simulink library "mfeval_STI_LIB"  (R2026a)
settings: Solver=ode45
undefined symbols (not defined in the file or in its folder): parameterStruct, userDynamics
libraries: sharedtransform x4, sharedutil x2, mfeval_CPI_LIB x1
Description:
  | Copyright 2020-2026 The MathWorks, Inc.
settings Model: Creator=MFURLANT  LastModifiedBy=smiller
settings DataIOCC: SaveFormat=StructureWithTime
settings HardwareCC: ProdHWDeviceType=Specified

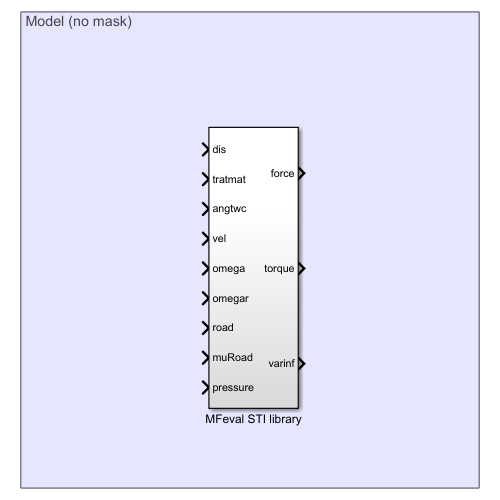
[thumbnail: Simulink's stored preview of the top-level diagram]
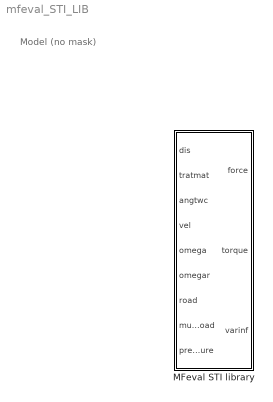
== system mfeval_STI_LIB ==
  note: Model (no mask)
  MFeval STI library : Subsystem

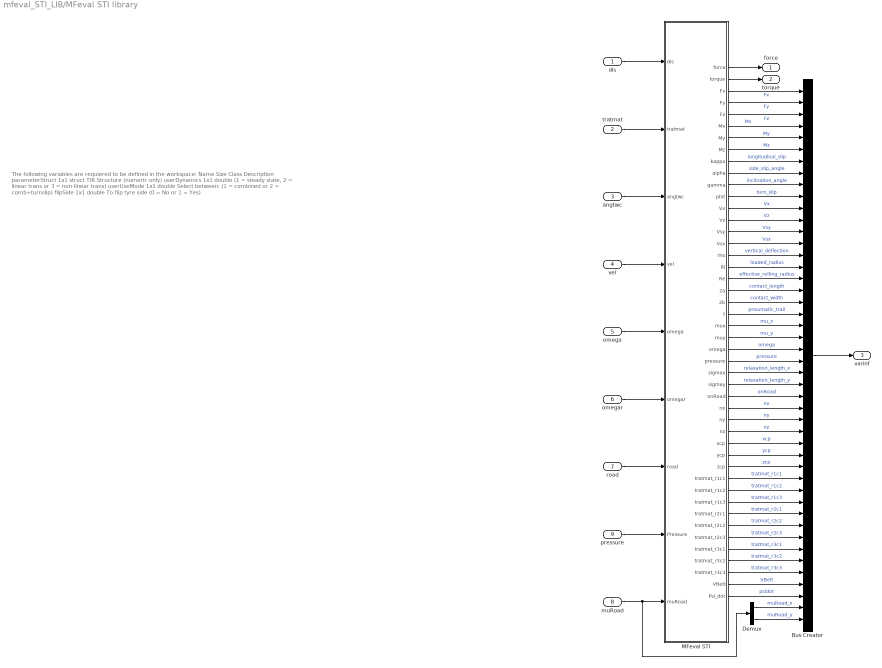
== system mfeval_STI_LIB/MFeval STI library ==
  note: The following variables are requiered to be defined in the workspace:
      |
      | Name
      | Size
      | Class
      | Description
      |
      | parameterStruct
      | 1x1
      | struct
      | TIR Structure (numeric only)
      |
      | userDynamics
      | 1x1
      | double
      | (1 = steady state, 2 = linear trans or 3 = non-linear trans)
      |
      | userUseMode
      | 1x1
      | double
      | Select between: (1 = combined or 2 = comb+turnslip)
      |
      | flipSide
      | 1x1
      | double
      | To flip tyre side (0 = No or 1 = Yes)
  dis : Inport
  tratmat : Inport  Port=2
  angtwc : Inport  Port=3
  vel : Inport  Port=4
  omega : Inport  Port=5
  omegar : Inport  Port=6
  road : Inport  Port=7
  muRoad : Inport  Port=8
  pressure : Inport  Port=9
  Bus Creator : BusCreator  Inputs=46
  Demux : Demux  Outputs=2
  MFeval STI : Subsystem
  force : Outport  VectorParamsAs1DForOutWhenUnconnected=off
  torque : Outport  Port=2  VectorParamsAs1DForOutWhenUnconnected=off
  varinf : Outport  Port=3  VectorParamsAs1DForOutWhenUnconnected=off
  wires:
  MFeval STI/7(My) -> Bus Creator/5  "My"
  MFeval STI/17(rho) -> Bus Creator/15  "vertical_deflection"
  MFeval STI/9(kappa) -> Bus Creator/7  "longitudinal_slip"
  MFeval STI/13(Vx) -> Bus Creator/11  "Vx"
  MFeval STI/8(Mz) -> Bus Creator/6  "Mz"
  MFeval STI/14(Vz) -> Bus Creator/12  "Vz"
  MFeval STI/10(alpha) -> Bus Creator/8  "side_slip_angle"
  MFeval STI/16(Vsx) -> Bus Creator/14  "Vsx"
  MFeval STI/1(force) -> force/1
  MFeval STI/2(torque) -> torque/1
  Bus Creator/1 -> varinf/1
  MFeval STI/3(Fx) -> Bus Creator/1  "Fx"
  MFeval STI/4(Fy) -> Bus Creator/2  "Fy"
  MFeval STI/5(Fz) -> Bus Creator/3  "Fz"
  MFeval STI/6(Mx) -> Bus Creator/4  "Mx"
  MFeval STI/19(Re) -> Bus Creator/17  "effective_rolling_radius"
  MFeval STI/15(Vsy) -> Bus Creator/13  "Vsy"
  MFeval STI/18(Rl) -> Bus Creator/16  "loaded_radius"
  MFeval STI/11(gamma) -> Bus Creator/9  "inclination_angle"
  MFeval STI/20(2a) -> Bus Creator/18  "contact_length"
  MFeval STI/27(sigmax) -> Bus Creator/25  "relaxation_length_x"
  MFeval STI/28(sigmay) -> Bus Creator/26  "relaxation_length_y"
  MFeval STI/23(mux) -> Bus Creator/21  "mu_x"
  MFeval STI/22(t) -> Bus Creator/20  "pneumatic_trail"
  MFeval STI/26(pressure) -> Bus Creator/24  "pressure"
  MFeval STI/12(phit) -> Bus Creator/10  "turn_slip"
  MFeval STI/24(muy) -> Bus Creator/22  "mu_y"
  MFeval STI/25("omega ") -> Bus Creator/23  "omega"
  MFeval STI/21(2b) -> Bus Creator/19  "contact_width"
  MFeval STI/29(onRoad) -> Bus Creator/27  "onRoad"
  MFeval STI/30(nx) -> Bus Creator/28  "nx"
  MFeval STI/31(ny) -> Bus Creator/29  "ny"
  MFeval STI/32(nz) -> Bus Creator/30  "nz"
  MFeval STI/33(xcp) -> Bus Creator/31  "xcp"
  MFeval STI/34(ycp) -> Bus Creator/32  "ycp"
  MFeval STI/35(zcp) -> Bus Creator/33  "zcp"
  MFeval STI/36(tratmat_r1c1) -> Bus Creator/34  "tratmat_r1c1"
  MFeval STI/37(tratmat_r1c2) -> Bus Creator/35  "tratmat_r1c2"
  MFeval STI/38(tratmat_r1c3) -> Bus Creator/36  "tratmat_r1c3"
  MFeval STI/39(tratmat_r2c1) -> Bus Creator/37  "tratmat_r2c1"
  MFeval STI/40(tratmat_r2c2) -> Bus Creator/38  "tratmat_r2c2"
  MFeval STI/41(tratmat_r2c3) -> Bus Creator/39  "tratmat_r2c3"
  MFeval STI/42(tratmat_r3c1) -> Bus Creator/40  "tratmat_r3c1"
  MFeval STI/43(tratmat_r3c2) -> Bus Creator/41  "tratmat_r3c2"
  MFeval STI/44(tratmat_r3c3) -> Bus Creator/42  "tratmat_r3c3"
  MFeval STI/45(VBelt) -> Bus Creator/43  "VBelt"
  MFeval STI/46(Psi_dot) -> Bus Creator/44  "psidot"
  muRoad/1 -> Demux/1, MFeval STI/9(muRoad)
  road/1 -> MFeval STI/7(road)
  omegar/1 -> MFeval STI/6(omegar)
  omega/1 -> MFeval STI/5(omega)
  vel/1 -> MFeval STI/4(vel)
  angtwc/1 -> MFeval STI/3(angtwc)
  tratmat/1 -> MFeval STI/2(tratmat)
  dis/1 -> MFeval STI/1(dis)
  pressure/1 -> MFeval STI/8(Pressure)
  Demux/1 -> Bus Creator/45  "muRoad_x"
  Demux/2 -> Bus Creator/46  "muRoad_y"

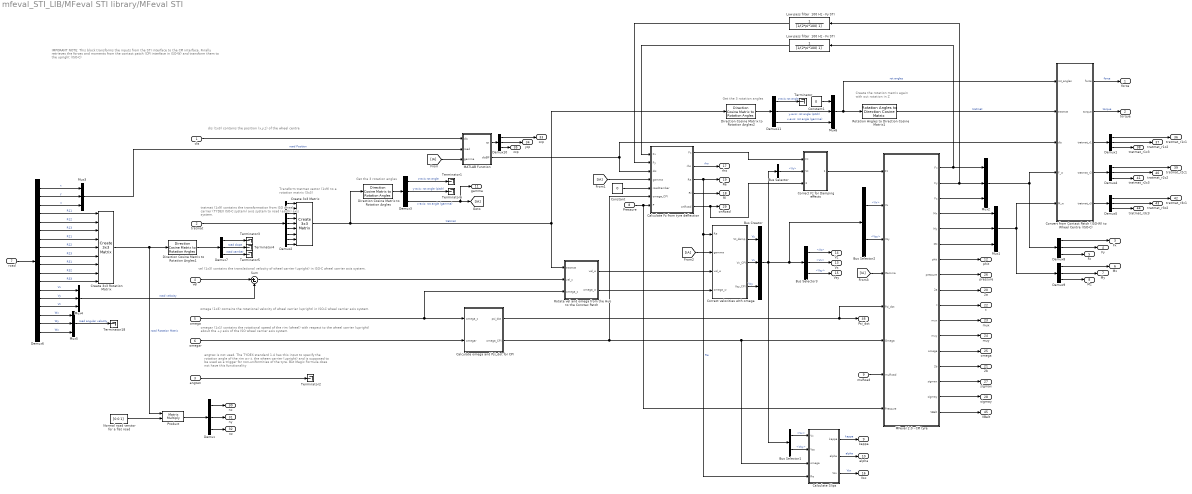
== system mfeval_STI_LIB/MFeval STI library/MFeval STI ==
  note: omegar (1x1) contains the rotational speed of the rim (wheel) with respect to the wheel carrier (upright) about the +y axis of the ISO wheel carrier axis system.
  note: omega (1x3) contains the rotational velocity of wheel carrier (upright) in ISO-C wheel carrier axis system.
  note: tratmat (1x9) contains the transformation from ISO wheel carrier (TYDEX ISO-C system) axis system to road (earth) axis system.
  note: vel (1x3) contains the translational velocity of wheel carrier (upright) in ISO-C wheel carrier axis system.
  note: IMPORANT NOTE:
      |
      | This block transforms the inputs from the STI interface to the CPI interface.
      | Finally retrieves the forces and moments from the contact patch (CPI interface in ISO-W) and transform them to the upright (ISO-C)
  note: angtwc is not used.
      | The TYDEX standard 1.4 has this input to specify the rotation angle of the rim w.r.t. the wheen carrier (upright) and is supposed to be used as a trigger for non-uniformities of the tyre. But Magic Formula does not have this functionality
  note: dis (1x3) contains the position (x,y,z) of the wheel centre
  note: Get the 3 rotation angles
  note: Transform tratmat vector (1x9)
      | to a rotation matrix (3x3)
  note: Create the rotation matrix again with out rotation in Z
  note: Get the 3 rotation angles
  dis : Inport
  tratmat : Inport  Port=2
  angtwc : Inport  Port=3
  vel : Inport  Port=4
  omega : Inport  Port=5
  omegar : Inport  Port=6
  road : Inport  Port=7
  Pressure : Inport  Port=8
  muRoad : Inport  Port=9
  Bus Creator : BusCreator  Inputs=3
  Bus Selector : BusSelector  OutputSignals=Vz
  Bus Selector1 : BusSelector  OutputSignals=Vx,Vsy
  Bus Selector2 : BusSelector  OutputSignals=Vx,Vsy
  Bus Selector3 : BusSelector  OutputSignals=Vz,Vx,Vsy
  Calculate Fz from tyre deflection : MATLAB Function  TreatAsAtomicUnit=on
  Calculate Slips : MATLAB Function  TreatAsAtomicUnit=on
  Calculate omega and Psi_dot for CPI : Subsystem
  Constant : Constant  Value=0
  Constant1 : Constant  Value=0
  Convert from Contact Patch (ISO-W) to Wheel Centre (ISO-C) : MATLAB Function  TreatAsAtomicUnit=on
  Correct Fz for Damping effects : Subsystem
  Correct velocities with omega : Subsystem
  Create 3x3 Matrix : sharedutil/Create 3x3 Matrix  aMode=aMode
  Create 3x3 Rotation Matrix : sharedutil/Create 3x3 Matrix  aMode=aMode
  Demux{,1,3..5,7..11} (10 alike) : Demux  Outputs=3
      Demux settings: DisplayOption=none
      Demux1 settings: DisplayOption=none
      Demux10 settings: DisplayOption=none
      Demux4 settings: DisplayOption=none
      Demux5 settings: DisplayOption=none
      Demux8 settings: DisplayOption=none
      Demux9 settings: DisplayOption=none
  Demux2 : Demux  Outputs=9
  Demux6 : Demux  Outputs=18
  Direction Cosine Matrix to Rotation Angles : sharedtransform/Direction Cosine Matrix to Rotation Angles  rotationOrder=ZYX  aMode=aMode  action=None  tolerance=eps(2)
  Direction Cosine Matrix to Rotation Angles1 : sharedtransform/Direction Cosine Matrix to Rotation Angles  rotationOrder=ZYX  aMode=aMode  action=None  tolerance=eps(2)
  Direction Cosine Matrix to Rotation Angles2 : sharedtransform/Direction Cosine Matrix to Rotation Angles  rotationOrder=ZYX  aMode=aMode  action=None  tolerance=eps(2)
  Low pass filter  100 Hz - Fx STI : TransferFcn  Denominator=[1/(2*pi*100) 1]
  Low pass filter  100 Hz - Fy STI : TransferFcn  Denominator=[1/(2*pi*100) 1]
  MATLAB Function : MATLAB Function  TreatAsAtomicUnit=on
  MFeval 2.0 - CPI tyre : Subsystem
  Mux{1..6} (6 alike) : Mux  Inputs=3
  Normal road verctor for a flat road : Constant  Value=[0 0 1]
  Product : Product  Multiplication=Matrix(*)
  Rotate vel and omega from the Hub to the Conctac Patch : Subsystem
  Rotation Angles to Direction Cosine Matrix1 : sharedtransform/Rotation Angles to Direction Cosine Matrix  rotationOrder=ZYX  aMode=aMode
  Sum : Sum  Inputs=|+-
  Terminator{,1..6,18} (8 alike) : Terminator
  force : Outport  VectorParamsAs1DForOutWhenUnconnected=off
  torque : Outport  Port=2  VectorParamsAs1DForOutWhenUnconnected=off
  Fx : Outport  Port=3  VectorParamsAs1DForOutWhenUnconnected=off
  Fy : Outport  Port=4  VectorParamsAs1DForOutWhenUnconnected=off
  Fz : Outport  Port=5  VectorParamsAs1DForOutWhenUnconnected=off
  Mx : Outport  Port=6  VectorParamsAs1DForOutWhenUnconnected=off
  My : Outport  Port=7  VectorParamsAs1DForOutWhenUnconnected=off
  Mz : Outport  Port=8  VectorParamsAs1DForOutWhenUnconnected=off
  kappa : Outport  Port=9  VectorParamsAs1DForOutWhenUnconnected=off
  alpha : Outport  Port=10  VectorParamsAs1DForOutWhenUnconnected=off
  gamma : Outport  Port=11  VectorParamsAs1DForOutWhenUnconnected=off
  phit : Outport  Port=12  VectorParamsAs1DForOutWhenUnconnected=off
  Vx : Outport  Port=13  VectorParamsAs1DForOutWhenUnconnected=off
  Vz : Outport  Port=14  VectorParamsAs1DForOutWhenUnconnected=off
  Vsy : Outport  Port=15  VectorParamsAs1DForOutWhenUnconnected=off
  Vsx : Outport  Port=16  VectorParamsAs1DForOutWhenUnconnected=off
  rho : Outport  Port=17  VectorParamsAs1DForOutWhenUnconnected=off
  Rl : Outport  Port=18  VectorParamsAs1DForOutWhenUnconnected=off
  Re : Outport  Port=19  VectorParamsAs1DForOutWhenUnconnected=off
  2a : Outport  Port=20  VectorParamsAs1DForOutWhenUnconnected=off
  2b : Outport  Port=21  VectorParamsAs1DForOutWhenUnconnected=off
  t : Outport  Port=22  VectorParamsAs1DForOutWhenUnconnected=off
  mux : Outport  Port=23  VectorParamsAs1DForOutWhenUnconnected=off
  muy : Outport  Port=24  VectorParamsAs1DForOutWhenUnconnected=off
  "omega " : Outport  Port=25  VectorParamsAs1DForOutWhenUnconnected=off
  pressure : Outport  Port=26  VectorParamsAs1DForOutWhenUnconnected=off
  sigmax : Outport  Port=27  VectorParamsAs1DForOutWhenUnconnected=off
  sigmay : Outport  Port=28  VectorParamsAs1DForOutWhenUnconnected=off
  onRoad : Outport  Port=29  VectorParamsAs1DForOutWhenUnconnected=off
  nx : Outport  Port=30  VectorParamsAs1DForOutWhenUnconnected=off
  ny : Outport  Port=31  VectorParamsAs1DForOutWhenUnconnected=off
  nz : Outport  Port=32  VectorParamsAs1DForOutWhenUnconnected=off
  xcp : Outport  Port=33  VectorParamsAs1DForOutWhenUnconnected=off
  ycp : Outport  Port=34  VectorParamsAs1DForOutWhenUnconnected=off
  zcp : Outport  Port=35  VectorParamsAs1DForOutWhenUnconnected=off
  tratmat_r1c1 : Outport  Port=36  VectorParamsAs1DForOutWhenUnconnected=off
  tratmat_r1c2 : Outport  Port=37  VectorParamsAs1DForOutWhenUnconnected=off
  tratmat_r1c3 : Outport  Port=38  VectorParamsAs1DForOutWhenUnconnected=off
  tratmat_r2c1 : Outport  Port=39  VectorParamsAs1DForOutWhenUnconnected=off
  tratmat_r2c2 : Outport  Port=40  VectorParamsAs1DForOutWhenUnconnected=off
  tratmat_r2c3 : Outport  Port=41  VectorParamsAs1DForOutWhenUnconnected=off
  tratmat_r3c1 : Outport  Port=42  VectorParamsAs1DForOutWhenUnconnected=off
  tratmat_r3c2 : Outport  Port=43  VectorParamsAs1DForOutWhenUnconnected=off
  tratmat_r3c3 : Outport  Port=44  VectorParamsAs1DForOutWhenUnconnected=off
  VBelt : Outport  Port=45  VectorParamsAs1DForOutWhenUnconnected=off
  Psi_dot : Outport  Port=46  VectorParamsAs1DForOutWhenUnconnected=off
  wires:
  Calculate Fz from tyre deflection/4(Rl) -> Rl/1
  angtwc/1 -> Terminator2/1
  MFeval 2.0 - CPI tyre/1(Fx) -> Low pass filter  100 Hz - Fx STI/1, Mux2/1
  MFeval 2.0 - CPI tyre/2(Fy) -> Low pass filter  100 Hz - Fy STI/1, Mux2/2
  tratmat/1 -> Demux2/1
  MFeval 2.0 - CPI tyre/4(Mx) -> Mux1/1
  MFeval 2.0 - CPI tyre/5(My) -> Mux1/2
  Mux1/1 -> Convert from Contact Patch (ISO-W) to Wheel Centre (ISO-C)/5(M_w), Demux9/1
  Mux2/1 -> Convert from Contact Patch (ISO-W) to Wheel Centre (ISO-C)/4(F_w), Demux8/1
  MFeval 2.0 - CPI tyre/3("Fz ") -> Mux2/3
  Demux3/1 -> Terminator1/1  "z-axis rot angle"
  Demux3/2 -> Terminator6/1  "y-axis: rot angle (pitch)"
  MATLAB Function/2(disEff) -> Calculate Fz from tyre deflection/3(dis), Convert from Contact Patch (ISO-W) to Wheel Centre (ISO-C)/3(dis)
  Create 3x3 Matrix/1 -> Direction Cosine Matrix to Rotation Angles/1, Rotate vel and omega from the Hub to the Conctac Patch/1(tratmat), Direction Cosine Matrix to Rotation Angles2/1  "tratmat"
  Convert from Contact Patch (ISO-W) to Wheel Centre (ISO-C)/1(force) -> force/1  "force"
  Convert from Contact Patch (ISO-W) to Wheel Centre (ISO-C)/2(torque) -> torque/1  "torque"
  Demux2/1 -> Create 3x3 Matrix/1
  Demux2/2 -> Create 3x3 Matrix/2
  Demux2/3 -> Create 3x3 Matrix/3
  Demux2/4 -> Create 3x3 Matrix/4
  Demux2/5 -> Create 3x3 Matrix/5
  Demux2/6 -> Create 3x3 Matrix/6
  Demux2/7 -> Create 3x3 Matrix/7
  Demux2/8 -> Create 3x3 Matrix/8
  Demux2/9 -> Create 3x3 Matrix/9
  omegar/1 -> Calculate omega and Psi_dot for CPI/2(omegar)
  Calculate Fz from tyre deflection/2(rho) -> rho/1  "rho"
  Calculate omega and Psi_dot for CPI/2(omega_CPI) -> Calculate Fz from tyre deflection/6(omega_CPI), MFeval 2.0 - CPI tyre/6(Omega), Calculate Slips/3(omega)
  Sum/1 -> Rotate vel and omega from the Hub to the Conctac Patch/2(vel_c)
  Calculate Fz from tyre deflection/1(Fz) -> Correct Fz for Damping effects/1(Fz)
  MFeval 2.0 - CPI tyre/6(Mz) -> Mux1/3
  MFeval 2.0 - CPI tyre/7(phit) -> phit/1
  MFeval 2.0 - CPI tyre/8(pressure) -> pressure/1
  MFeval 2.0 - CPI tyre/9(2a) -> 2a/1
  MFeval 2.0 - CPI tyre/10(t) -> t/1
  MFeval 2.0 - CPI tyre/11(mux) -> mux/1
  MFeval 2.0 - CPI tyre/12(muy) -> muy/1
  MFeval 2.0 - CPI tyre/13(omega) -> "omega "/1
  MFeval 2.0 - CPI tyre/14(2b) -> 2b/1
  MFeval 2.0 - CPI tyre/15(sigmax) -> sigmax/1
  MFeval 2.0 - CPI tyre/16(sigmay) -> sigmay/1
  Rotate vel and omega from the Hub to the Conctac Patch/1(vel_w) -> Correct velocities with omega/3(vel_w)
  Rotate vel and omega from the Hub to the Conctac Patch/2(omega_w) -> Correct velocities with omega/4(omega_w)
  Calculate Slips/1(kappa) -> kappa/1  "kappa"
  Calculate Slips/2(alpha) -> alpha/1  "alpha"
  Calculate Slips/3(Vsx) -> Vsx/1  "Vsx"
  Calculate Fz from tyre deflection/3(Re) -> Calculate Slips/4(Re), Correct velocities with omega/1(Re), Re/1  "Re"
  Correct velocities with omega/1(Vz_damp) -> Bus Creator/1  "Vz"
  Correct velocities with omega/2(Vx_CPI) -> Bus Creator/2  "Vx"
  Correct velocities with omega/3(Vsy_CPI) -> Bus Creator/3  "Vsy"
  Bus Creator/1 -> Bus Selector1/1, Bus Selector2/1, Bus Selector3/1, Bus Selector/1
  Bus Selector/1 -> Correct Fz for Damping effects/2(Vz)  "<Vz>"
  Bus Selector1/1 -> Calculate Slips/1(Vx)  "<Vx>"
  Bus Selector1/2 -> Calculate Slips/2(Vsy)  "<Vsy>"
  Bus Selector2/1 -> MFeval 2.0 - CPI tyre/2(Vx)  "<Vx>"
  Bus Selector2/2 -> MFeval 2.0 - CPI tyre/3(Vsy)  "<Vsy>"
  Bus Selector3/3 -> Vsy/1  "<Vsy>"
  Bus Selector3/2 -> Vx/1  "<Vx>"
  Bus Selector3/1 -> Vz/1  "<Vz>"
  Low pass filter  100 Hz - Fy STI/1 -> Calculate Fz from tyre deflection/2(Fy)
  Low pass filter  100 Hz - Fx STI/1 -> Calculate Fz from tyre deflection/1(Fx)
  Demux10/1 -> xcp/1
  Demux10/2 -> ycp/1
  Demux10/3 -> zcp/1
  Convert from Contact Patch (ISO-W) to Wheel Centre (ISO-C)/3(tratmat_r1) -> Demux1/1
  Convert from Contact Patch (ISO-W) to Wheel Centre (ISO-C)/4(tratmat_r2) -> Demux4/1
  Convert from Contact Patch (ISO-W) to Wheel Centre (ISO-C)/5(tratmat_r3) -> Demux5/1
  Demux1/1 -> tratmat_r1c1/1
  Demux1/2 -> tratmat_r1c2/1
  Demux1/3 -> tratmat_r1c3/1
  Demux4/1 -> tratmat_r2c1/1
  Demux4/2 -> tratmat_r2c2/1
  Demux4/3 -> tratmat_r2c3/1
  Demux5/1 -> tratmat_r3c1/1
  Demux5/2 -> tratmat_r3c2/1
  Demux5/3 -> tratmat_r3c3/1
  MFeval 2.0 - CPI tyre/17(VBelt) -> VBelt/1
  road/1 -> Demux6/1
  Demux6/1 -> Mux3/1  "x"
  Demux6/2 -> Mux3/2  "y"
  Demux6/3 -> Mux3/3  "z"
  Demux6/4 -> Create 3x3 Rotation Matrix/1  "R11"
  Demux6/5 -> Create 3x3 Rotation Matrix/2  "R12"
  Demux6/6 -> Create 3x3 Rotation Matrix/3  "R13"
  Demux6/7 -> Create 3x3 Rotation Matrix/4  "R21"
  Demux6/8 -> Create 3x3 Rotation Matrix/5  "R22"
  Demux6/9 -> Create 3x3 Rotation Matrix/6  "R23"
  Demux6/10 -> Create 3x3 Rotation Matrix/7  "R31"
  Demux6/11 -> Create 3x3 Rotation Matrix/8  "R32"
  Demux6/12 -> Create 3x3 Rotation Matrix/9  "R33"
  Demux6/13 -> Mux4/1  "Vx"
  Demux6/14 -> Mux4/2  "Vy"
  Demux6/15 -> Mux4/3  "Vz"
  Demux6/16 -> Mux5/1  "Wx"
  Demux6/17 -> Mux5/2  "Wy"
  Demux6/18 -> Mux5/3  "Wz"
  Mux3/1 -> MATLAB Function/2(road)  "road Position"
  Mux4/1 -> Sum/2  "road velocity"
  Create 3x3 Rotation Matrix/1 -> Product/1, Direction Cosine Matrix to Rotation Angles1/1  "road Rotation Matrix"
  Direction Cosine Matrix to Rotation Angles1/1 -> Demux7/1
  Demux7/1 -> Terminator3/1
  Demux7/2 -> Terminator4/1  "road slope"
  Demux3/3 -> gamma/1, [IA]  "x-axis: rot angle (gamma)"
  Demux7/3 -> Terminator5/1  "road camber"
  Demux8/1 -> Fx/1
  Demux8/2 -> Fy/1
  Demux8/3 -> Fz/1
  Demux9/1 -> Mx/1
  Demux9/2 -> My/1
  Demux9/3 -> Mz/1
  Demux/2 -> ny/1
  Demux/3 -> nz/1
  Demux/1 -> nx/1
  Product/1 -> Demux/1
  Normal road verctor for a flat road/1 -> Product/2
  Constant/1 -> Calculate Fz from tyre deflection/5(roadCamber)
  dis/1 -> MATLAB Function/1(dis)
  Mux5/1 -> Terminator18/1  "road angular velocity"
  MATLAB Function/1(cp) -> Demux10/1
  vel/1 -> Sum/1
  muRoad/1 -> MFeval 2.0 - CPI tyre/7(muRoad)
  Demux11/2 -> Mux6/2  "y-axis: rot angle (pitch)"
  Mux6/1 -> Convert from Contact Patch (ISO-W) to Wheel Centre (ISO-C)/1(rot_angles), Rotation Angles to Direction Cosine Matrix1/1  "rot angles"
  Demux11/3 -> Mux6/3  "x-axis: rot angle (gamma)"
  Direction Cosine Matrix to Rotation Angles2/1 -> Demux11/1
  Demux11/1 -> Terminator/1  "z-axis rot angle"
  Rotation Angles to Direction Cosine Matrix1/1 -> Convert from Contact Patch (ISO-W) to Wheel Centre (ISO-C)/2(tratmat)  "tratmat"
  [IA] -> MATLAB Function/3(gamma)
  [IA] -> Calculate Fz from tyre deflection/4(gamma)
  [IA] -> Correct velocities with omega/2(gamma)
  [IA] -> MFeval 2.0 - CPI tyre/4(Gamma)
  Calculate Fz from tyre deflection/5(onRoad) -> onRoad/1, Correct Fz for Damping effects/3(onRoad)
  Correct Fz for Damping effects/1(Fz_CPI) -> MFeval 2.0 - CPI tyre/1(Fz)
  Direction Cosine Matrix to Rotation Angles/1 -> Demux3/1
  Constant1/1 -> Mux6/1
  Pressure/1 -> MFeval 2.0 - CPI tyre/8(Pressure), Calculate Fz from tyre deflection/7(P)
  omega/1 -> Rotate vel and omega from the Hub to the Conctac Patch/3(omega_c), Calculate omega and Psi_dot for CPI/1(omega_c)
  Calculate omega and Psi_dot for CPI/1(psi_dot) -> MFeval 2.0 - CPI tyre/5(Psi_dot), Psi_dot/1

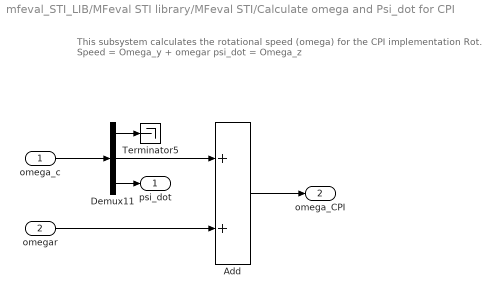
== system mfeval_STI_LIB/MFeval STI library/MFeval STI/Calculate omega and Psi_dot for CPI ==
  note: This subsystem calculates the rotational speed (omega) for the CPI implementation
      |
      | Rot. Speed = Omega_y + omegar
      | psi_dot = Omega_z
  omega_c : Inport
  omegar : Inport  Port=2
  Add : Sum
  Demux11 : Demux  Outputs=3
      settings: DisplayOption=none
  Terminator5 : Terminator
  psi_dot : Outport  VectorParamsAs1DForOutWhenUnconnected=off
  omega_CPI : Outport  Port=2  VectorParamsAs1DForOutWhenUnconnected=off
  wires:
  Add/1 -> omega_CPI/1
  omega_c/1 -> Demux11/1
  omegar/1 -> Add/2
  Demux11/1 -> Terminator5/1
  Demux11/3 -> psi_dot/1
  Demux11/2 -> Add/1

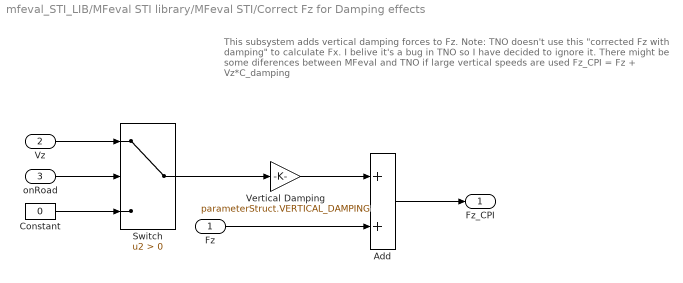
== system mfeval_STI_LIB/MFeval STI library/MFeval STI/Correct Fz for Damping effects ==
  note: This subsystem adds vertical damping forces to Fz.
      |
      | Note: TNO doesn't use this "corrected Fz with damping" to calculate Fx.
      | I belive it's a bug in TNO so I have decided to ignore it.
      | There might be some diferences between MFeval and TNO if large vertical speeds are used
      |
      |
      | Fz_CPI = Fz + Vz*C_damping
  Fz : Inport
  Vz : Inport  Port=2
  onRoad : Inport  Port=3
  Add : Sum
  Constant : Constant  Value=0
  Switch : Switch  Criteria=u2 > Threshold  SaturateOnIntegerOverflow=off  InputSameDT=off
  Vertical Damping : Gain  Gain=parameterStruct.VERTICAL_DAMPING
  Fz_CPI : Outport  VectorParamsAs1DForOutWhenUnconnected=off
  wires:
  Fz/1 -> Add/2
  Add/1 -> Fz_CPI/1
  Vz/1 -> Switch/1
  Vertical Damping/1 -> Add/1
  onRoad/1 -> Switch/2
  Constant/1 -> Switch/3
  Switch/1 -> Vertical Damping/1

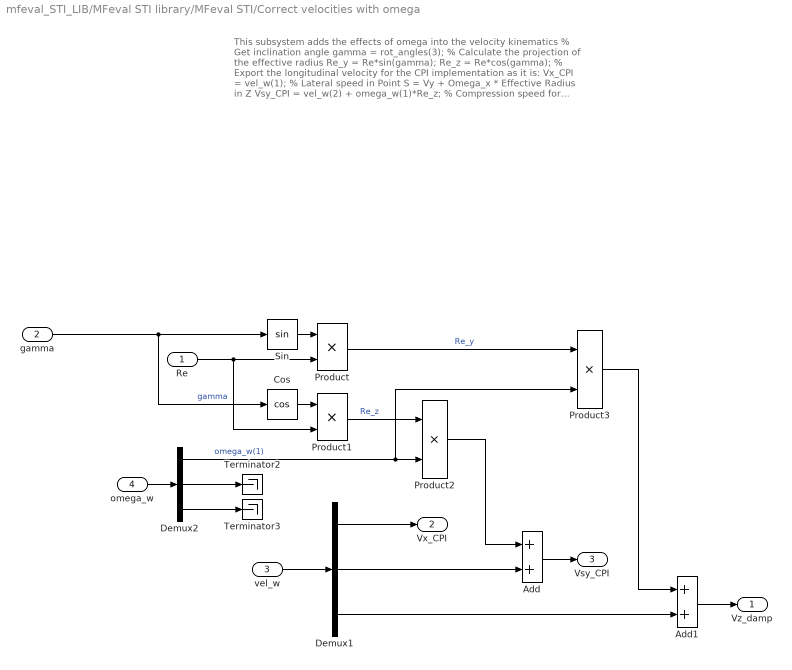
== system mfeval_STI_LIB/MFeval STI library/MFeval STI/Correct velocities with omega ==
  note: This subsystem adds the effects of omega into the velocity kinematics
      |
      | % Get inclination angle
      | gamma = rot_angles(3);
      |
      | % Calculate the projection of the effective radius
      | Re_y = Re*sin(gamma);
      | Re_z = Re*cos(gamma);
      |
      | % Export the longitudinal velocity for the CPI implementation as it is:
      | Vx_CPI = vel_w(1);
      |
      | % Lateral speed in Point S = Vy + Omega_x * Effective Radius in Z
      | Vsy_CPI = vel_w(2) + omega_w(1)*Re_z;
      |
      | % Compression speed for damping effects:
      | Vz_damp = vel_w(3) + omega_w(1)*Re_y;
  Re : Inport
  gamma : Inport  Port=2
  vel_w : Inport  Port=3
  omega_w : Inport  Port=4
  Add : Sum
  Add1 : Sum
  Cos : Trigonometry  Operator=cos
  Demux1 : Demux  Outputs=3
      settings: DisplayOption=none
  Demux2 : Demux  Outputs=3
      settings: DisplayOption=none
  Product{,1..3} (4 alike) : Product
  Sin : Trigonometry
  Terminator2 : Terminator
  Terminator3 : Terminator
  Vz_damp : Outport  VectorParamsAs1DForOutWhenUnconnected=off
  Vx_CPI : Outport  Port=2  VectorParamsAs1DForOutWhenUnconnected=off
  Vsy_CPI : Outport  Port=3  VectorParamsAs1DForOutWhenUnconnected=off
  wires:
  gamma/1 -> Sin/1, Cos/1  "gamma"
  Sin/1 -> Product/1
  Re/1 -> Product1/2, Product/2
  Cos/1 -> Product1/1
  Product/1 -> Product3/1  "Re_y"
  Product1/1 -> Product2/1  "Re_z"
  vel_w/1 -> Demux1/1
  Demux1/1 -> Vx_CPI/1
  Demux1/2 -> Add/2
  omega_w/1 -> Demux2/1
  Demux2/3 -> Terminator3/1
  Demux2/2 -> Terminator2/1
  Demux2/1 -> Product3/2, Product2/2  "omega_w(1)"
  Product2/1 -> Add/1
  Add/1 -> Vsy_CPI/1
  Product3/1 -> Add1/1
  Demux1/3 -> Add1/2
  Add1/1 -> Vz_damp/1

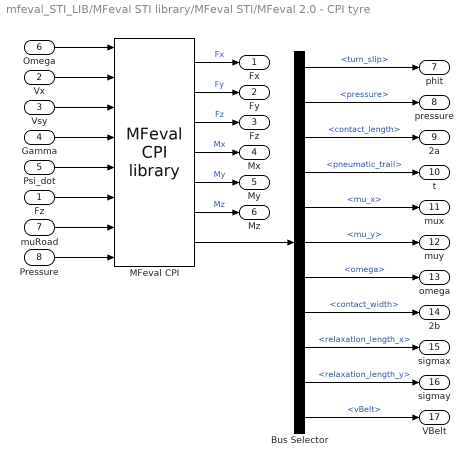
== system mfeval_STI_LIB/MFeval STI library/MFeval STI/MFeval 2.0 - CPI tyre ==
  Fz : Inport
  Vx : Inport  Port=2
  Vsy : Inport  Port=3
  Gamma : Inport  Port=4
  Psi_dot : Inport  Port=5
  Omega : Inport  Port=6
  muRoad : Inport  Port=7
  Pressure : Inport  Port=8
  Bus Selector : BusSelector  OutputSignals=turn_slip,pressure,contact_length,pneumatic_trail,mu_x,mu_y,omega,contact_width,relaxation_length_x,relaxation_length_y,vBelt
  MFeval CPI : mfeval_CPI_LIB/MFeval CPI library  SystemSampleTime=-1  VariantActivationTime=update diagram  EmptyChoice=off  PassThrough=off  PassThroughVariantControl=(default)  EmptyChoiceVariantControl=(default)  AllowFlexibleInterface=on  Latency=0  AutoFrameSizeCalculation=off
  Fx : Outport  VectorParamsAs1DForOutWhenUnconnected=off
  Fy : Outport  Port=2  VectorParamsAs1DForOutWhenUnconnected=off
  "Fz " : Outport  Port=3  VectorParamsAs1DForOutWhenUnconnected=off
  Mx : Outport  Port=4  VectorParamsAs1DForOutWhenUnconnected=off
  My : Outport  Port=5  VectorParamsAs1DForOutWhenUnconnected=off
  Mz : Outport  Port=6  VectorParamsAs1DForOutWhenUnconnected=off
  phit : Outport  Port=7  VectorParamsAs1DForOutWhenUnconnected=off
  pressure : Outport  Port=8  VectorParamsAs1DForOutWhenUnconnected=off
  2a : Outport  Port=9  VectorParamsAs1DForOutWhenUnconnected=off
  t : Outport  Port=10  VectorParamsAs1DForOutWhenUnconnected=off
  mux : Outport  Port=11  VectorParamsAs1DForOutWhenUnconnected=off
  muy : Outport  Port=12  VectorParamsAs1DForOutWhenUnconnected=off
  omega : Outport  Port=13  VectorParamsAs1DForOutWhenUnconnected=off
  2b : Outport  Port=14  VectorParamsAs1DForOutWhenUnconnected=off
  sigmax : Outport  Port=15  VectorParamsAs1DForOutWhenUnconnected=off
  sigmay : Outport  Port=16  VectorParamsAs1DForOutWhenUnconnected=off
  VBelt : Outport  Port=17  VectorParamsAs1DForOutWhenUnconnected=off
  wires:
  Omega/1 -> MFeval CPI/1
  Vx/1 -> MFeval CPI/2
  Vsy/1 -> MFeval CPI/3
  Gamma/1 -> MFeval CPI/4
  Psi_dot/1 -> MFeval CPI/5
  MFeval CPI/1 -> Fx/1  "Fx"
  MFeval CPI/2 -> Fy/1  "Fy"
  MFeval CPI/3 -> "Fz "/1  "Fz"
  MFeval CPI/4 -> Mx/1  "Mx"
  MFeval CPI/5 -> My/1  "My"
  MFeval CPI/6 -> Mz/1  "Mz"
  Bus Selector/2 -> pressure/1  "<pressure>"
  Bus Selector/1 -> phit/1  "<turn_slip>"
  Bus Selector/7 -> omega/1  "<omega>"
  Bus Selector/8 -> 2b/1  "<contact_width>"
  Bus Selector/3 -> 2a/1  "<contact_length>"
  Bus Selector/4 -> t/1  "<pneumatic_trail>"
  Bus Selector/5 -> mux/1  "<mu_x>"
  Bus Selector/6 -> muy/1  "<mu_y>"
  Bus Selector/9 -> sigmax/1  "<relaxation_length_x>"
  Bus Selector/10 -> sigmay/1  "<relaxation_length_y>"
  Bus Selector/11 -> VBelt/1  "<vBelt>"
  Fz/1 -> MFeval CPI/6
  MFeval CPI/7 -> Bus Selector/1
  muRoad/1 -> MFeval CPI/7
  Pressure/1 -> MFeval CPI/8

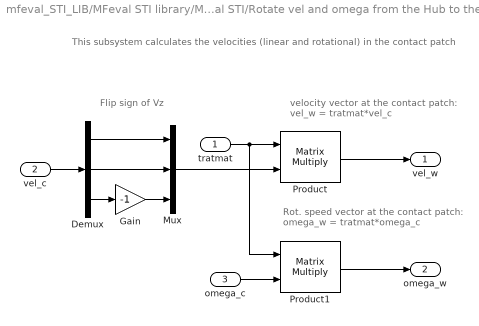
== system mfeval_STI_LIB/MFeval STI library/MFeval STI/Rotate vel and omega from the Hub to the Conctac Patch ==
  note: Rot. speed vector at the contact patch:
      | omega_w = tratmat*omega_c
  note: Flip sign of Vz
  note: velocity vector at the contact patch:
      | vel_w = tratmat*vel_c
  note: This subsystem calculates the velocities (linear and rotational) in the contact patch
  tratmat : Inport
  vel_c : Inport  Port=2
  omega_c : Inport  Port=3
  Demux : Demux  Outputs=3
      settings: DisplayOption=none
  Gain : Gain  Gain=-1
  Mux : Mux  Inputs=3
  Product : Product  Multiplication=Matrix(*)
  Product1 : Product  Multiplication=Matrix(*)
  vel_w : Outport  VectorParamsAs1DForOutWhenUnconnected=off
  omega_w : Outport  Port=2  VectorParamsAs1DForOutWhenUnconnected=off
  wires:
  vel_c/1 -> Demux/1
  Demux/1 -> Mux/1
  Demux/3 -> Gain/1
  Demux/2 -> Mux/2
  Mux/1 -> Product/2
  tratmat/1 -> Product1/1, Product/1
  Product/1 -> vel_w/1
  omega_c/1 -> Product1/2
  Product1/1 -> omega_w/1
  Gain/1 -> Mux/3

== matlab function mfeval_STI_LIB/MFeval STI library/MFeval STI/MATLAB Function ==
  data: dis input; road input; cp output; gamma input; disEff output
function [cp, disEff] = fcn(dis, road, gamma)

% Effective distance
disEff = dis;
disEff(3) = disEff(3)-road(3);

% Contact Point coordinates
cp = dis;
cp(2) = dis(2) + (dis(3)/tan(pi/2-gamma));
cp(3) = road(3);

== matlab function mfeval_STI_LIB/MFeval STI library/MFeval STI/Calculate Slips ==
  data: parameterStruct parameter; Vx input; Vsy input; omega input; Re input; kappa output; alpha output; Vsx output
function [kappa, alpha, Vsx]  = fcn(parameterStruct, Vx, Vsy, omega, Re)
%#codegen

% This function calculates the slip inputs without damping effects. 
% Note that these slip inputs are not used in the CPI calculations. 
% This is how TNO has implemented the calculations, so here we are
% doing the same...


% Longitudinal slip velocity
Vsx = Vx - Re.*omega; % [Eqn (2.3) Page 64 - Book]

% Check if is low speed
isLowSpeed = abs(Vx) < parameterStruct.VXLOW;

if isLowSpeed
    % Avoid sign(0) = 0
    signVx = sign(Vx);
    signVx(signVx == 0) = 1;
   
    % Low speed Slip Ratio Calculation
    kappa = -(Vsx) * signVx;
else
    % Slip Ratio Calculation
    kappa = -(Vsx./Vx); % [Eqn (2.4) Page 64 - Book]
end

if isnan(kappa)
    kappa = 0;
end

% Slip Angle
alpha = atan(Vsy./abs(Vx)); % [Eqn (2.9) Page 67 - Book]

% Important Note:
% Due to the ISO sign convention, equation 2.9 does not need a
% negative sign. The pacejka book is written in adapted SAE.

if isnan(alpha)
    alpha = 0;
end

== matlab function mfeval_STI_LIB/MFeval STI library/MFeval STI/Calculate Fz from tyre deflection ==
  data: parameterStruct parameter; Fx input; Fy input; dis input; gamma input; roadCamber input; Fz output; omega_CPI input; P input; rho output; Re output; Rl output; userDynamics parameter; onRoad output
function [Fz, rho, Re, Rl, onRoad] = fcn(parameterStruct, Fx, Fy, dis, gamma, roadCamber, omega_CPI, P, userDynamics)
%#codegen


% This function calculates the Fz from the tyre deflection

%[MODEL]
Vo      = parameterStruct.LONGVL               ; %Nominal speed
pio     = parameterStruct.NOMPRES              ; %Reference pressure

%[VERTICAL]
Fzo     = parameterStruct.FNOMIN         		; %Nominal wheel load
Cz0     = parameterStruct.VERTICAL_STIFFNESS	; %Tyre vertical stiffness
Q_RE0	= parameterStruct.Q_RE0       			; %Ratio of free tyre radius with nominal tyre radius
Q_V1	= parameterStruct.Q_V1  				; %Tyre radius increase with speed
Q_V2	= parameterStruct.Q_V2    				; %Vertical stiffness increase with speed
Q_FZ2	= parameterStruct.Q_FZ2      			; %Quadratic term in load vs. deflection
PFZ1	= parameterStruct.PFZ1    				; %Pressure effect on vertical stiffness
Q_FCX    = parameterStruct.Q_FCX;
Q_FCY    = parameterStruct.Q_FCY;

BREFF   = parameterStruct.BREFF      			; %Low load stiffness effective rolling radius
DREFF	= parameterStruct.DREFF     			; %Peak value of effective rolling radius
FREFF	= parameterStruct.FREFF    			; %High load stiffness effective rolling radius

BOTTOM_OFFST = parameterStruct.BOTTOM_OFFST    ; %Distance to rim when bottoming starts to occur
BOTTOM_STIFF = parameterStruct.BOTTOM_STIFF    ; %Vertical stiffness of bottomed tyre

%[DIMENSION]
Ro          = parameterStruct.UNLOADED_RADIUS      ; %Free tyre radius
RIM_RADIUS  = parameterStruct.RIM_RADIUS          ; %Nominal rim radius

% Loaded Radius [m]
Rl = dis(3)/cos(gamma);

% Normalized change in inflation pressure
dpi = (P - pio)./pio; % [Eqn (4.E2b) Page 177 - Book]

% Free-spinning radius
Romega = Ro .* (Q_RE0 + Q_V1.*((omega_CPI.*Ro)./Vo).^2); % [Eqn (1) Page 2 - Paper] - Centrifugal growth of the free tyre radius

% Nominal stiffness (pressure corrected)
Cz = Cz0 .* (1 + PFZ1.*dpi); % [Eqn (5) Page 2 - Paper] - Vertical stiffness adapted for tyre inflation pressure

% Tyre deflection
rhoz0 = max((Romega-Rl),0);

rho = rhoz0/cos(-roadCamber);

% Model parameters as QFZ1 that normally aren't present in the TIR files
Q_FZ1 = sqrt((Cz0.*Ro./Fzo).^2 - 4.* Q_FZ2); % Rearranging [Eqn (4) Page 2 - Paper]

if userDynamics == 1
    % Calculate Fz without external effects
    Fz = (1 + Q_V2*(Ro/Vo)*abs(omega_CPI))*(Q_FZ1*(rho/Ro)+ Q_FZ2*(rho/Ro)^2)*(1+PFZ1*dpi)*Fzo; % [Eqn (3) Page 2 - Paper]
else
    if parameterStruct.FITTYP == 61
        % Calculate Fz with MF6.1 equations
        Fz = (1 + Q_V2*(Ro/Vo)*abs(omega_CPI)-(Q_FCX*Fx/Fzo)^2-(Q_FCY*Fy/Fzo)^2)*(Q_FZ1*(rho/Ro)+ Q_FZ2*(rho/Ro)^2)*(1+PFZ1*dpi)*Fzo; % [Eqn (3) Page 2 - Paper]
    else
        solver = mfeval.Solver;
        [Fz, rho] = solver.calculateFz62(parameterStruct, gamma, omega_CPI, Romega, dpi, Rl, Fx, Fy);
    end
end

% Variable to determine if there is wheel lift
if rho == 0
    onRoad = 0;
else
    onRoad = 1;
end

% Bottoming model:
Fz_btm = BOTTOM_STIFF * (RIM_RADIUS+BOTTOM_OFFST-Rl); %Equation on page 22 of the TNO Equation Manual (Bottoming model)
Fz = max(Fz, Fz_btm); %Equation on page 23 of the TNO Equation Manual (Bottoming model)

% Effective Rolling Radius
Re = Romega -(Fzo./Cz) .* ( DREFF .*atan( BREFF.*(Fz./Fzo)) + FREFF.*(Fz./Fzo)); % [Eqn (7) Page 2 - Paper]

== matlab function mfeval_STI_LIB/MFeval STI library/MFeval STI/Convert from Contact Patch (ISO-W) to Wheel Centre (ISO-C) ==
  data: rot_angles input; tratmat input; dis input; force output; torque output; F_w input; M_w input; tratmat_r1 output; tratmat_r2 output; tratmat_r3 output
function [force, torque, tratmat_r1, tratmat_r2,tratmat_r3]= fcn(rot_angles, tratmat, dis, F_w, M_w)
%#codegen

% This function rotates and translates forces and moments from the 
% contact patch to the wheel centre

% Get angles
pitch = rot_angles(2);

% Rotation of forces and moments:
force = tratmat*F_w;
M_c = tratmat*M_w;

% Pre assign variable torque
torque = zeros(3,1);

% Calculate deltas
deltaZ = dis(3);
deltaX = tan(pitch)*deltaZ;


% Translation of moments:
torque(1) = M_c(1) + force(2)*deltaZ;

torque(2) = M_c(2) - force(1)*deltaZ - force(3)*deltaX ;

torque(3) = M_c(3)+ force(2)*deltaX;

% Export transformation matrix rows
tratmat_r1 = tratmat(1,:)';
tratmat_r2 = tratmat(2,:)';
tratmat_r3 = tratmat(3,:)';
